simulink model "SystemWithFuzzyLogic"  (R2023a)
settings: Solver=VariableStepAuto  StartTime=0.0  StopTime=50  MaxStep=0.1  RelTol=1e-2  AbsTol=1e-2  EnableMultiTasking=on
libraries: fuzblock x1, simulink x1
settings Model: Creator=KozlovM  LastModifiedBy=diontep
settings SolverCC: AutoScaleAbsTol=off  AlgebraicLoopSolver=TrustRegion  MaxZcPerStep=1
settings DataIOCC: LimitDataPoints=on  MaxDataPoints=10000
settings OptimizationCC: ReuseModelBlockBuffer=off  LifeSpan=inf
settings DebuggingCC: UnconnectedInputMsg=warning  UnconnectedOutputMsg=warning  UnconnectedLineMsg=warning  AllowSymbolicDim=off  SubsystemReferenceDiagnosticForUnitTest=warning  SFUnexpectedBacktrackingDiag=warning  SFNoUnconditionalDefaultTransitionDiag=warning  SFExecutionAtInitializationDiag=none  ArithmeticOperatorsInVariantConditions=warning
settings ModelReferenceCC: EnableRefExpFcnMdlSchedulingChecks=on
settings SFSimCC: SimUseLocalCustomCode=off  CustomCodeUndefinedFunction=UseInterfaceOnly
settings RTWCC: RTWUseLocalCustomCode=off  DLArmComputeVersion=19.05
settings CodeAppCC: StateflowObjectComments=on
settings GRTTargetCC: TargetLangStandard=C89/C90 (ANSI)
settings ConfigComp: CovMetricSettings=dw  CovSaveCumulativeToWorkspaceVar=on  CovSaveSingleToWorkspaceVar=on  CovExternalEMLEnable=off  CovSFcnEnable=off
settings SimscapeCC: SimscapeLogType=all  SimscapeLogSimulationStatistics=on  SimscapeLogDataHistory=10000

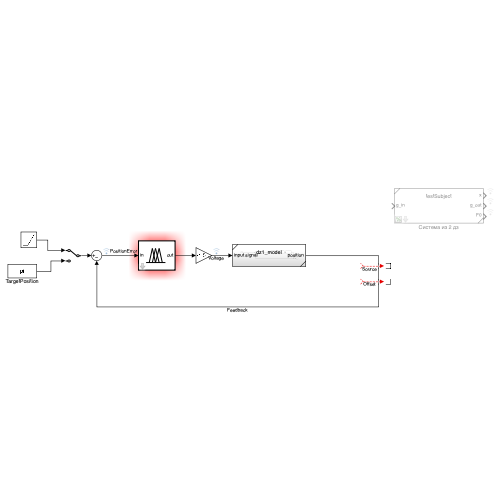
[thumbnail: Simulink's stored preview of the top-level diagram]
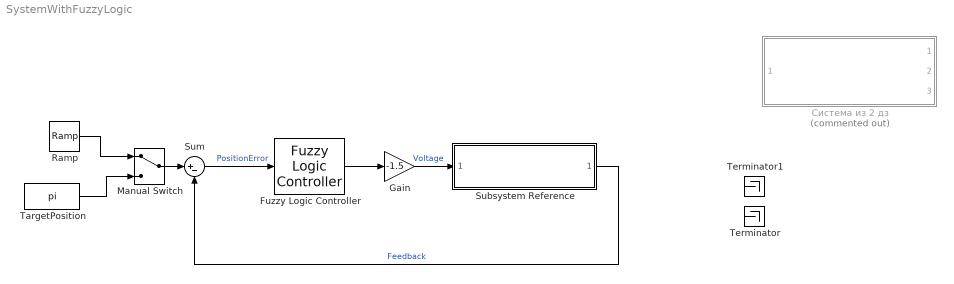
== system SystemWithFuzzyLogic ==
  Fuzzy Logic Controller : fuzblock/Fuzzy Logic  Controller  FIS=inverted_pendulum  OutputSampleNumber=101  DataType=double  FuzzifiedInputs=off  RuleFiringStrengths=off  RuleOutputs=off  AggregatedOutputs=off  SimulateUsing=Interpreted execution  OutOfRangeInputValueMessage=warning  NoRuleFiredMessage=warning  EmptyOutputFuzzySetMessage=warning
  Gain : Gain  Gain=-1.5
  Manual Switch : ManualSwitch
  Ramp : simulink/Sources/Ramp  slope=1  start=0  InitialOutput=0
  Subsystem Reference : Subsystem  ReferencedSubsystem=dz1_model
  Sum : Sum  Inputs=|+-
  TargetPosition : Constant  Value=pi
  Terminator : Terminator
  Terminator1 : Terminator
  Система из 2 дз : Subsystem  Commented=on  ReferencedSubsystem=testSubject
  wires:
  Fuzzy Logic Controller/1 -> Gain/1
  Sum/1 -> Fuzzy Logic Controller/1  "PositionError"
  Subsystem Reference/1 -> Sum/2  "Feedback"
  Ramp/1 -> Manual Switch/1
  Manual Switch/1 -> Sum/1
  TargetPosition/1 -> Manual Switch/2
  Gain/1 -> Subsystem Reference/1  "Voltage"
  ? -> Terminator/1  "Offset"
  ? -> Terminator1/1  "Source"
